simulink model "ram"  (R2020a)
settings: Solver=VariableStepAuto  StartTime=0.0  StopTime=inf  RelTol=1e-3
libraries: hdlsllib x1
settings Model: Creator=F1  LastModifiedBy=F1

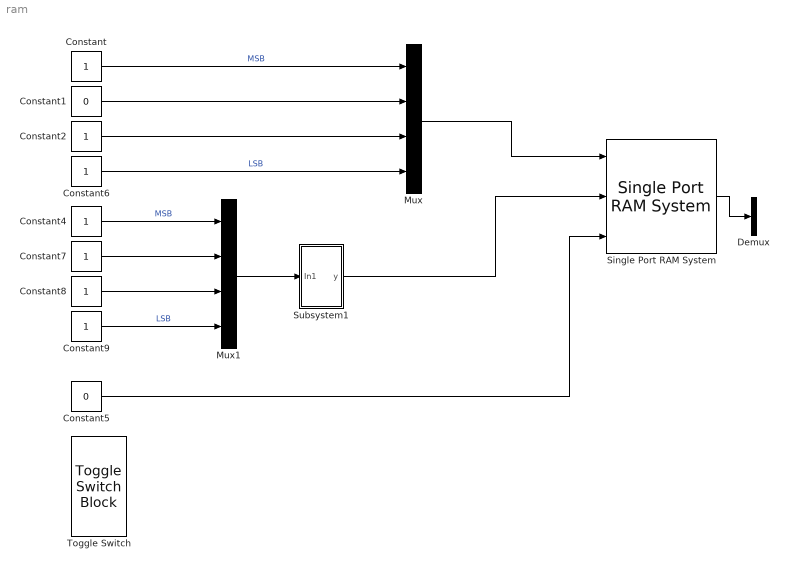
== system ram ==
  Constant{,2,4,6..9} (7 alike) : Constant
  Constant1 : Constant  Value=0
  Constant5 : Constant  Value=0
  Demux : Demux
  Mux : Mux
  Mux1 : Mux
  Single Port RAM System : hdlsllib/HDL RAMs/Single Port RAM System  RAMType=Single port  WriteOutputValue=New data  RAMInitialValue=0  SimulateUsing=Code generation
      settings: SourceProductBaseCode=SL
  Subsystem1 : Subsystem
  Toggle Switch : ToggleSwitchBlock
      settings: Values={{'Off', 'On'}, [0 1]}
  wires:
  Constant5/1 -> Single Port RAM System/3
  Constant/1 -> Mux/1  "MSB"
  Constant1/1 -> Mux/2
  Constant2/1 -> Mux/3
  Constant6/1 -> Mux/4  "LSB"
  Mux/1 -> Single Port RAM System/1
  Constant4/1 -> Mux1/1  "MSB"
  Constant9/1 -> Mux1/4  "LSB"
  Constant7/1 -> Mux1/2
  Constant8/1 -> Mux1/3
  Mux1/1 -> Subsystem1/1(In1)
  Subsystem1/1(y) -> Single Port RAM System/2
  Single Port RAM System/1 -> Demux/1

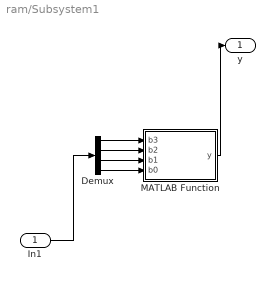
== system ram/Subsystem1 ==
  In1 : Inport
  Demux : Demux
  MATLAB Function : MATLAB Function  TreatAsAtomicUnit=on
  y : Outport
  wires:
  Demux/3 -> MATLAB Function/3(b1)
  Demux/1 -> MATLAB Function/1(b3)
  Demux/2 -> MATLAB Function/2(b2)
  Demux/4 -> MATLAB Function/4(b0)
  MATLAB Function/1(y) -> y/1
  In1/1 -> Demux/1

== matlab function ram/Subsystem1/MATLAB Function ==
  data: b3 input; y output; b2 input; b1 input; b0 input
function y = fcn( b3   , b2   , b1    , b0    )
y =  b3*2^3 + b2*2^2 + b1*2^1 + b0*2^0 ;
end
